simulink model "SIL3"  (R2024b)
settings: Solver=VariableStepAuto  StartTime=0.0  StopTime=10.0  RelTol=1e-3
values from neighbouring files (symbols this model uses):
  b = 7.2e-5    (= 7.2e-05)    [HIL.m]    (also in SIL.m = 4.2697318139e-06)
  g = 9.81    [HIL.m]    (also in SIL.m)
  L = 0.42e-3    (= 0.00042)    [HIL.m]    (also in SIL.m)
  M = J/L^2    (= 23.4693877551)    [SIL.m]
settings Model: Creator=tclaverie303  LastModifiedBy=julien.dbc

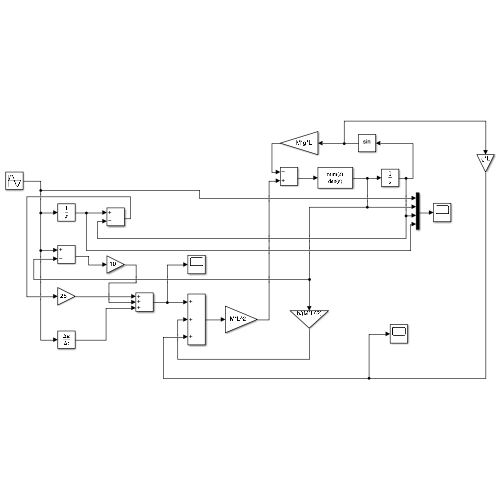
[thumbnail: Simulink's stored preview of the top-level diagram]
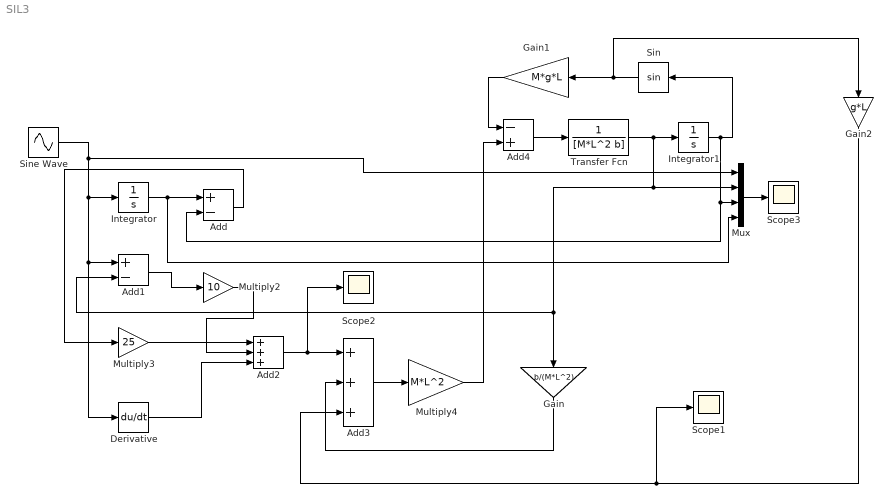
== system SIL3 ==
  Add : Sum  Inputs=+-
  Add1 : Sum  Inputs=+-
  Add2 : Sum  Inputs=+++
  Add3 : Sum  Inputs=+++
  Add4 : Sum  Inputs=-+
  Derivative : Derivative
  Gain : Gain  Gain=b/(M*L^2)
  Gain1 : Gain  Gain=M*g*L
  Gain2 : Gain  Gain=g*L
  Integrator : Integrator
  Integrator1 : Integrator
  Multiply2 : Gain  Gain=10
  Multiply3 : Gain  Gain=25
  Multiply4 : Gain  Gain=M*L^2
  Mux : Mux
  Scope1 : Scope
  Scope2 : Scope
  Scope3 : Scope
  Sin : Trigonometry
  Sine Wave : Sin  SampleTime=0
  Transfer Fcn : TransferFcn  Denominator=[M*L^2 b]
  wires:
  Add/1 -> Multiply3/1
  Add1/1 -> Multiply2/1
  Sine Wave/1 -> Mux/1, Add1/1, Derivative/1, Integrator/1
  Add3/1 -> Multiply4/1
  Derivative/1 -> Add2/3
  Multiply2/1 -> Add2/2
  Multiply3/1 -> Add2/1
  Integrator/1 -> Mux/4, Add/1
  Add2/1 -> Scope2/1, Add3/1
  Gain/1 -> Add3/2
  Gain1/1 -> Add4/1
  Multiply4/1 -> Add4/2
  Transfer Fcn/1 -> Mux/2, Add1/2, Gain/1, Integrator1/1
  Add4/1 -> Transfer Fcn/1
  Mux/1 -> Scope3/1
  Sin/1 -> Gain2/1, Gain1/1
  Integrator1/1 -> Mux/3, Add/2, Sin/1
  Gain2/1 -> Scope1/1, Add3/3
